simulink model "Encoder_reader_simulink"  (R2025a)
settings: Solver=FixedStepAuto  StartTime=0.0  StopTime=inf  FixedStep=0.1  RelTol=1e-3  EnableMultiTasking=on
libraries: stm32f4xxblockslib x3, stm32g4xxblockslib x3
settings Model: STM32="{\"EncoderBlockForG4\":[{\"ID\":\"untitled:1\"},{\"ID\":\"Lab3_Encoder:1\"},{\"ID\":\"Encoder_reader_simulink:42\"},{\"ID\":\"Encoder_reader_simulink:1\"},{\"ID\":\"Encoder_reader_simulink:33\"}],\"DigitalPortRead\":[{\"ID\":\"Encoder_reader_simulink:49\"},{\"ID\":\"Encoder_reader_simulink:46\"},{\"ID\":\"Encoder_reader_simulink:47\"}]}"  SimulationMode=external  PacingRate=10  Creator=User  LastModifiedBy=User
settings OptimizationCC: DefaultParameterBehavior=Inlined  EnhancedBackFolding=on  PassReuseOutputArgsAs=Individual arguments  ZeroExternalMemoryAtStartup=off  ZeroInternalMemoryAtStartup=off  MaxStackSize=512  OptimizeBlockOrder=speed  DifferentSizesBufferReuse=on  OptimizationCustomize=off  EfficientTunableParamExpr=on
settings DebuggingCC: ParameterTunabilityLossMsg=error
settings HardwareCC: ProdBitPerPointer=32.0  ProdBitPerSizeT=32.0  ProdBitPerPtrDiffT=32.0  ProdLargestAtomicInteger=Long  ProdLargestAtomicFloat=Double  ProdWordSize=32.0  ProdLongLongMode=on  ProdHWDeviceType=ARM Compatible->ARM Cortex-M
settings SFSimCC: MATLABDynamicMemAlloc=off
settings RTWCC: SystemTargetFile=ert.tlc  HardwareBoard=STM32G4xx Based  TemplateMakefile=ert_default_tmf  Toolchain=GNU Tools for ARM Embedded Processors  Description=Embedded Coder
settings CodeAppCC: ForceParamTrailComments=on  IgnoreCustomStorageClasses=off  OperatorAnnotations=on  SimulinkDataObjDesc=on  SFDataObjDesc=on  InsertBlockDesc=on
settings ERTTargetCC: ExtModeTransport=3.0  ExtModeStaticAllocSize=2048.0  TargetLangStandard=C99 (ISO)  CodeReplacementLibrary=ARM Cortex-M  SupportContinuousTime=on

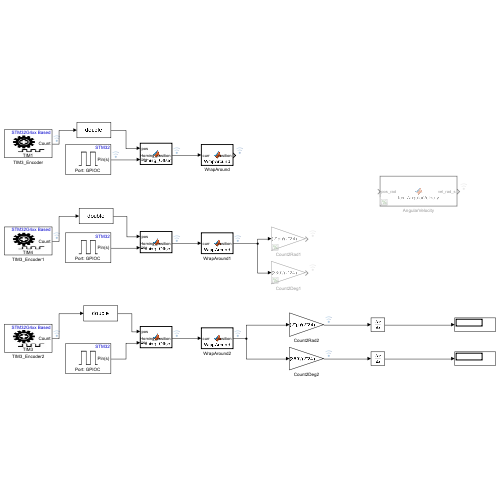
[thumbnail: Simulink's stored preview of the top-level diagram]
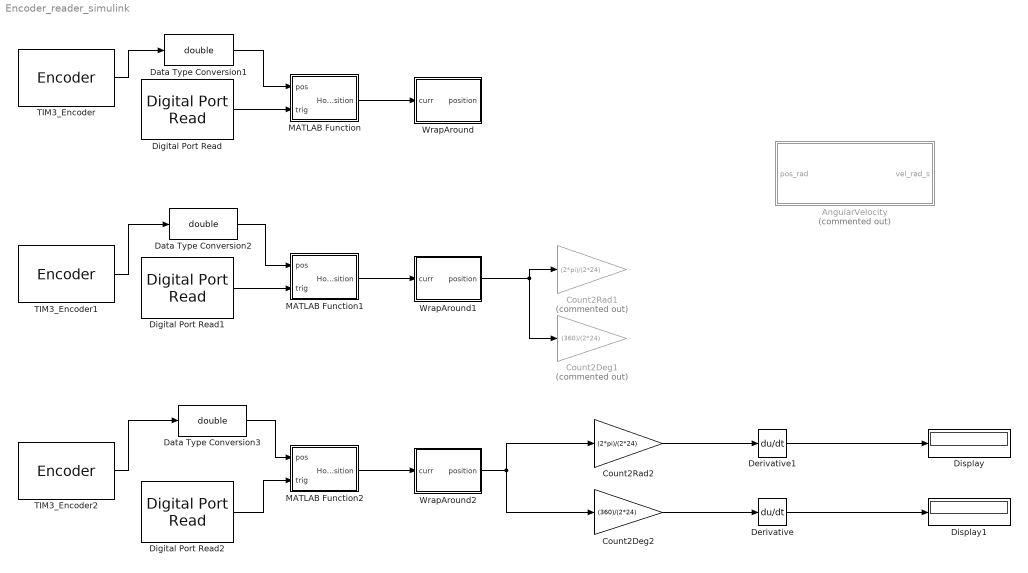
== system Encoder_reader_simulink ==
  AngularVelocity : MATLAB Function  Commented=on  TreatAsAtomicUnit=on
  Count2Deg1 : Gain  Commented=on  Gain=(360)/(2*24)
  Count2Deg2 : Gain  Gain=(360)/(2*24)
  Count2Rad1 : Gain  Commented=on  Gain=(2*pi)/(2*24)
  Count2Rad2 : Gain  Gain=(2*pi)/(2*24)
  Data Type Conversion1 : DataTypeConversion  OutDataTypeStr=double  SaturateOnIntegerOverflow=off  RndMeth=Floor
  Data Type Conversion2 : DataTypeConversion  OutDataTypeStr=double  SaturateOnIntegerOverflow=off  RndMeth=Floor
  Data Type Conversion3 : DataTypeConversion  OutDataTypeStr=double  SaturateOnIntegerOverflow=off  RndMeth=Floor
  Derivative : Derivative
  Derivative1 : Derivative
  Digital Port Read : stm32f4xxblockslib/Digital Port Read  PortName=GPIOC  PinNumber=[13]  ReadOperation=on  IOAsArray=on  SampleTime=-1  EnableSimPort=off  hoistedMaskSrc=ECSoC/ECSimCodegen/Digital Port Read
  Digital Port Read1 : stm32f4xxblockslib/Digital Port Read  PortName=GPIOC  PinNumber=[13]  ReadOperation=on  IOAsArray=on  SampleTime=-1  EnableSimPort=off  hoistedMaskSrc=ECSoC/ECSimCodegen/Digital Port Read
  Digital Port Read2 : stm32f4xxblockslib/Digital Port Read  PortName=GPIOC  PinNumber=[13]  ReadOperation=on  IOAsArray=on  SampleTime=-1  EnableSimPort=off  hoistedMaskSrc=ECSoC/ECSimCodegen/Digital Port Read
  Display : Display
  Display1 : Display
  MATLAB Function : MATLAB Function  TreatAsAtomicUnit=on
  MATLAB Function1 : MATLAB Function  TreatAsAtomicUnit=on
  MATLAB Function2 : MATLAB Function  TreatAsAtomicUnit=on
  TIM3_Encoder : stm32g4xxblockslib/Encoder  TimerModule=TIM1  EnableResetInput=off  OutputCountAfterFirstIndex=off  OutputValidIndex=off  OutputDirection=off  OutputStatus=off  SampleTime=-1
  TIM3_Encoder1 : stm32g4xxblockslib/Encoder  TimerModule=TIM4  EnableResetInput=off  OutputCountAfterFirstIndex=off  OutputValidIndex=off  OutputDirection=off  OutputStatus=off  SampleTime=-1
  TIM3_Encoder2 : stm32g4xxblockslib/Encoder  TimerModule=TIM3  EnableResetInput=off  OutputCountAfterFirstIndex=off  OutputValidIndex=off  OutputDirection=off  OutputStatus=off  SampleTime=-1
  WrapAround : MATLAB Function  TreatAsAtomicUnit=on
  WrapAround1 : MATLAB Function  TreatAsAtomicUnit=on
  WrapAround2 : MATLAB Function  TreatAsAtomicUnit=on
  wires:
  TIM3_Encoder/1 -> Data Type Conversion1/1
  Data Type Conversion1/1 -> MATLAB Function/1(pos)
  Data Type Conversion2/1 -> MATLAB Function1/1(pos)
  WrapAround1/1(position) -> Count2Rad1/1, Count2Deg1/1
  TIM3_Encoder1/1 -> Data Type Conversion2/1
  Data Type Conversion3/1 -> MATLAB Function2/1(pos)
  WrapAround2/1(position) -> Count2Deg2/1, Count2Rad2/1
  TIM3_Encoder2/1 -> Data Type Conversion3/1
  Digital Port Read/1 -> MATLAB Function/2(trig)
  Digital Port Read2/1 -> MATLAB Function2/2(trig)
  Digital Port Read1/1 -> MATLAB Function1/2(trig)
  MATLAB Function/1(Homing_position) -> WrapAround/1(curr)
  MATLAB Function1/1(Homing_position) -> WrapAround1/1(curr)
  MATLAB Function2/1(Homing_position) -> WrapAround2/1(curr)
  Count2Deg2/1 -> Derivative/1
  Count2Rad2/1 -> Derivative1/1
  Derivative/1 -> Display1/1
  Derivative1/1 -> Display/1

== matlab function Encoder_reader_simulink/WrapAround ==
  data: curr input; position output
function position = WrapAround(curr)
%#codegen
persistent last offset
if isempty(last)
    last = curr;
    offset = 0;
end

MAX_COUNT = 61439;
diff = double(curr) - double(last);

% ตรวจจับ overflow/underflow อย่างปลอดภัย
if diff >  MAX_COUNT/2
    offset = offset - (MAX_COUNT + 1);
elseif diff < -MAX_COUNT/2
    offset = offset + (MAX_COUNT + 1);
end

% ป้องกันกรณี spike ใหญ่ที่ไม่ใช่ overflow
if abs(diff) > MAX_COUNT*0.9
    diff = 0;
end

position = double(curr) + offset;
last = curr;
end

== matlab function Encoder_reader_simulink/WrapAround2 ==
  data: curr input; position output
function position = WrapAround(curr)
%#codegen
persistent last offset
if isempty(last)
    last = curr;
    offset = 0;
end

MAX_COUNT = 61439;
diff = double(curr) - double(last);

% ตรวจจับ overflow/underflow อย่างปลอดภัย
if diff >  MAX_COUNT/2
    offset = offset - (MAX_COUNT + 1);
elseif diff < -MAX_COUNT/2
    offset = offset + (MAX_COUNT + 1);
end

% ป้องกันกรณี spike ใหญ่ที่ไม่ใช่ overflow
if abs(diff) > MAX_COUNT*0.9
    diff = 0;
end

position = double(curr) + offset;
last = curr;
end

== matlab function Encoder_reader_simulink/MATLAB Function ==
  data: pos input; Homing_position output; trig input
function Homing_position = Homing_Offset(pos, trig)
%#codegen
persistent offset
if isempty(offset), offset = 0; end

% trigger = 1 → ตั้ง home ใหม่
if trig
    offset = pos;
end

% คืนค่าตำแหน่งสัมพัทธ์จาก home
Homing_position = pos - offset;
end

== matlab function Encoder_reader_simulink/MATLAB Function1 ==
  data: pos input; Homing_position output; trig input
function Homing_position = Homing_Offset(pos, trig)
%#codegen
persistent offset
if isempty(offset), offset = 0; end

% trigger = 1 → ตั้ง home ใหม่
if trig
    offset = pos;
end

% คืนค่าตำแหน่งสัมพัทธ์จาก home
Homing_position = pos - offset;
end

== matlab function Encoder_reader_simulink/MATLAB Function2 ==
  data: pos input; Homing_position output; trig input
function Homing_position = Homing_Offset(pos, trig)
%#codegen
persistent offset
if isempty(offset), offset = 0; end

% trigger = 1 → ตั้ง home ใหม่
if trig
    offset = pos;
end

% คืนค่าตำแหน่งสัมพัทธ์จาก home
Homing_position = pos - offset;
end

== matlab function Encoder_reader_simulink/AngularVelocity ==
  data: pos_rad input; vel_rad_s output
function vel_rad_s = fcn_AngularVelocity(pos_rad)
%#codegen
%
% คำนวณความเร็วเชิงมุม (rad/s)
% โดยการหาอนุพันธ์ของตำแหน่งเชิงมุม (rad) เทียบกับเวลา

% ---------------------------------------------------------
% !!! สำคัญ: ตั้งค่า Sample Time (Ts) !!!
%
% ค่านี้ต้องตรงกับ Sample Time ของ Simulink model ของคุณ
% (เช่น 0.001 สำหรับ 1ms, หรือ 0.01 สำหรับ 10ms)
Ts = 0.001; % <--- *** แก้ไขค่านี้ให้ถูกต้อง ***
% ---------------------------------------------------------

% ใช้ 'persistent' เพื่อจำค่าตำแหน่งของรอบที่แล้ว
persistent last_pos_rad;

% 1. กำหนดค่าเริ่มต้นเมื่อรันครั้งแรก
if isempty(last_pos_rad)
    last_pos_rad = pos_rad;
    % สำหรับรอบแรกสุด ให้ความเร็วเป็น 0
    vel_rad_s = 0.0;
else
    % 2. คำนวณ Delta (การเปลี่ยนแปลงตำแหน่ง)
    delta_pos = pos_rad - last_pos_rad;

    % 3. คำนวณ Velocity (rad/s)
    vel_rad_s = delta_pos / Ts;
end

% 4. เก็บค่าตำแหน่งปัจจุบันไว้สำหรับรอบถัดไป
last_pos_rad = pos_rad;

end

== matlab function Encoder_reader_simulink/WrapAround1 ==
  data: curr input; position output
function position = WrapAround(curr)
%#codegen
persistent last offset
if isempty(last)
    last = curr;
    offset = 0;
end

MAX_COUNT = 61439;
diff = double(curr) - double(last);

% ตรวจจับ overflow/underflow อย่างปลอดภัย
if diff >  MAX_COUNT/2
    offset = offset - (MAX_COUNT + 1);
elseif diff < -MAX_COUNT/2
    offset = offset + (MAX_COUNT + 1);
end

% ป้องกันกรณี spike ใหญ่ที่ไม่ใช่ overflow
if abs(diff) > MAX_COUNT*0.9
    diff = 0;
end

position = double(curr) + offset;
last = curr;
end
